simulink library "rappid_564xl_ec_toolbox"  (Simulink 8.1)
settings: Solver=FixedStepDiscrete  StartTime=0.0  StopTime=10.0  RelTol=1e-3
undefined symbols (not defined in the file or in its folder): CTU_unit, mem_AddrLW, mem_AddrUP, rappid_564xl_adc_input_support_rev2, rappid_564xl_can_support_rev2, read_mem_AddrLW, read_mem_AddrUP
(part 5 of 5)

== system rappid_564xl_ec_toolbox/MPC564xL/RAppID_564xL_Config ==

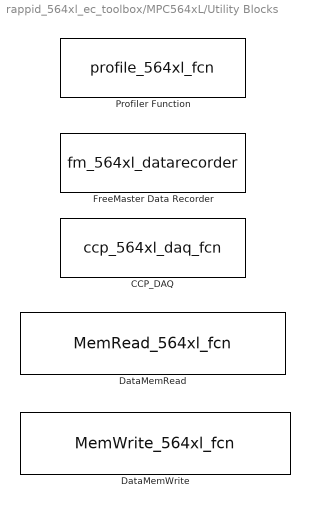
== system rappid_564xl_ec_toolbox/MPC564xL/Utility Blocks ==
  CCP_DAQ : S-Function  FunctionName=ccp_564xl_daq_fcn  Parameters=ccp_daq  EnableBusSupport=off  mask(ccp_daq_564xL_Func){ccp_daq=0}
      mask prompts: ccp_daq "Select the DAQ"
      mask help: CCP DAQ function - Place this block in a model to create DAQ trigger for CCP DAQ mode.
      mask Help: web([rappid_block_help,filesep,'ccp_daq.htm']);
      mask TypeOptions ccp_daq: 0 | 1 | 2 | 3 | 4 | 5 | 6 | 7 | 8 | 9 | 10 | 11 | 12 | 13 | 14 | 15 | 16 | 17 | 18 | 19 | 20 | 21 | 22 | 23 | 24 | 25 | 26 | 27 | 28 | 29 | 30 | 31 | 32 | 33 | 34 | 35 | 36 | 37 | 38 | 39 | 40 | 41 | 42 | 43 | 44 | 45 | 46 | 47 | 48 | 49 | 50 | 51 | 52 | 53 | 54 | 55 | 56 | 57 | 58 | 59 | 60 | 61 | 62 | 63 | 64 | 65 | 66 | 67 | 68 | 69 | 70 | 71 | 72 | 73 | 74 | 75 | 76 | 77 | 78 | 79 | 80 | 81 | 82 | 83 | 84 | 85 | 86 | 87 | 88 | 89 | 90 | 91 | 92 | 93 | 94 | 95 | 96 | 97 | 98 | 99 | 100 | 101 | 102 | 103 | 104 | 105 | 106 | 107 | 108 | 109 | 110 | 111 | 112 | 113 | 114 | 115 | 116 | 117 | 118 | 119 | 120 | 121 | 122 | 123 | 124 | 125 | 126 | 127 | 128 | 129 | 130 | 131 | 132 | 133 | 134 | 135 | 136 | 137 | 138 | 139 | 140 | 141 | 142 | 143 | 144 | 145 | 146 | 147 | 148 | 149 | 150 | 151 | 152 | 153 | 154 | 155 | 156 | 157 | 158 | 159 | 160 | 161 | 162 | 163 | 164 | 165 | 166 | 167 | 168 | 169 | 170 | 171 | 172 | 173 | 174 | 175 | 176 | 177 | 178 | 179 | 180 | 181 | 182 | 183 | 184 | 185 | 186 | 187 | 188 | 189 | 190 | 191 | 192 | 193 | 194 | 195 | 196 | 197 | 198 | 199 | 200 | 201 | 202 | 203 | 204 | 205 | 206 | 207 | 208 | 209 | 210 | 211 | 212 | 213 | 214 | 215 | 216 | 217 | 218 | 219 | 220 | 221 | 222 | 223 | 224 | 225 | 226 | 227 | 228 | 229 | 230 | 231 | 232 | 233 | 234 | 235 | 236 | 237 | 238 | 239 | 240 | 241 | 242 | 243 | 244 | 245 | 246 | 247 | 248 | 249 | 250 | 251 | 252 | 253 | 254 | 255
      mask Display: disp(['CCP DAQ : ',get_param(gcb,'ccp_daq')])
  DataMemRead : S-Function  FunctionName=MemRead_564xl_fcn  Parameters=uint16(read_mem_AddrUP),uint16(read_mem_AddrLW)  EnableBusSupport=off  mask(MemoryReadBlock){base_address=40000000, offset=C, ba=1073741824, off=12}
      mask prompts: base_address "Enter base address (e.f...0x20000000)"; offset "Enter Offset from base Address (e.g. ..0x4)"; off "Mask Parameter 4:"
      mask help: This block provides direct access to memory by address and offset into any memory section the processor has access. This block provides a direct memory read from the specified memory location.
      mask init:
      | mem = hex2dec(get_param(gcb,'base_address'));
      | off = hex2dec(get_param(gcb,'offset'));
      | memAddr = dec2hex(mem+off);
      | read_mem_Addr = hex2dec(memAddr);
      | set_param(gcb,'ba',num2str(mem));
      | set_param(gcb,'off',num2str(off));
      | memReadStr = ['Data Memory Read ',sprintf('\n'),'Address : 0x',memAddr,sprintf('\n')];
      mask Help: web([rappid_block_help,filesep,'Memory_Read.htm']);
      mask Callback offset:
      | mem = hex2dec(get_param(gcb,'base_address'));
      | off = hex2dec(get_param(gcb,'offset'));
      | memAddr = dec2hex(mem+off);
      | read_mem_AddrUP = hex2dec(memAddr(1:4));
      | read_mem_AddrLW = hex2dec(memAddr(5:8));
      | mem_Addr = hex2dec(memAddr);
      | 
      | if( mod(mem_Addr,4)>0)
      | 
      | error('Address needs to be within 32bit boundary')
      | 
      | end
      mask Display:
      | port_label('output',1,'Output Signal');
      | 
      | disp(memReadStr);
  DataMemWrite : S-Function  FunctionName=MemWrite_564xl_fcn  Parameters=uint16(mem_AddrUP),uint16(mem_AddrLW)  EnableBusSupport=off  mask(MemoryWriteBlock){base_address=40000000, offset=C, ba=1073741824, off=12}
      mask prompts: base_address "Enter base address (e.f...0x20000000)"; offset "Enter Offset from base Address (e.g. ..0x4)"; off "Mask Parameter 4:"
      mask help: This block provides direct access to memory by address and offset into any memory section the processor has access. This block allows a direct write to the specified memory location.
      mask init:
      | mem = hex2dec(get_param(gcb,'base_address'));
      | off = hex2dec(get_param(gcb,'offset'));
      | memAddr = dec2hex(mem+off);
      | mem_Addr = hex2dec(memAddr);
      | set_param(gcb,'ba',num2str(mem));
      | set_param(gcb,'off',num2str(off));
      | memWriteStr = ['Data Memory Write ',sprintf('\n'),'Address : 0x',memAddr,sprintf('\n')];
      mask Help: web([rappid_block_help,filesep,'Memory_Write.htm']);
      mask Callback offset:
      | mem = hex2dec(get_param(gcb,'base_address'));
      | off = hex2dec(get_param(gcb,'offset'));
      | memAddr = dec2hex(mem+off);
      | mem_AddrUP = hex2dec(memAddr(1:4));
      | mem_AddrLW = hex2dec(memAddr(5:8));
      | mem_Addr = hex2dec(memAddr);
      | 
      | if( mod(mem_Addr,4)>0)
      | 
      | error('Address needs to be within 32bit boundary')
      | 
      | end
      mask Display:
      | port_label('input',1,'Input Signal');
      | 
      | disp(memWriteStr);
  FreeMaster Data Recorder : S-Function  FunctionName=fm_564xl_datarecorder  EnableBusSupport=off  mask(fm_564xL_datarecorder){}
      mask help: This block allows the user to store variables in internal memory and download them through FreeMaster tool.
      mask Help: web([rappid_block_help,filesep,'fm_data_recorder.htm']);
      mask Display: disp(['FreeMaster Data Recorder'])
  "Profiler Function " : S-Function  Priority=1  FunctionName=profile_564xl_fcn  Parameters=profile_indx,showOut  EnableBusSupport=off  mask(Profile_564xL_Func){profile_indx=0, showOut=off}
      mask prompts: profile_indx "Select the profile Index"; showOut "Show Profile Output"
      mask help: Profile Function - Place this block in a model to profile the execution time of the function. This block places profiling code at the begining and end of the function this block is placed in. Select the index for this block-up to 100 blocks may be profiled at once so a profile index must be selected for each block.
      mask Help: web([rappid_block_help,filesep,'profile_function.htm']);
      mask TypeOptions profile_indx: 0 | 1 | 2 | 3 | 4 | 5 | 6 | 7 | 8 | 9 | 10 | 11 | 12 | 13 | 14 | 15 | 16 | 17 | 18 | 19 | 20 | 21 | 22 | 23 | 24 | 25 | 26 | 27 | 28 | 29 | 30 | 31 | 32 | 33 | 34 | 35 | 36 | 37 | 38 | 39 | 40 | 41 | 42 | 43 | 44 | 45 | 46 | 47 | 48 | 49 | 50 | 51 | 52 | 53 | 54 | 55 | 56 | 57 | 58 | 59 | 60 | 61 | 62 | 63 | 64 | 65 | 66 | 67 | 68 | 69 | 70 | 71 | 72 | 73 | 74 | 75 | 76 | 77 | 78 | 79 | 80 | 81 | 82 | 83 | 84 | 85 | 86 | 87 | 88 | 89 | 90 | 91 | 92 | 93 | 94 | 95 | 96 | 97 | 98 | 99
      mask Display: disp(['Profile Function Index : ',get_param(gcb,'profile_indx')])
